simulink model "notch_filters"  (R2014a)
settings: Solver=ode45  StartTime=0.0  StopTime=10.0  RelTol=1e-3
undefined symbols (not defined in the file): A1_notch_cmd, A1_notch_cmd_s, A2_notch_cmd, A2_notch_cmd_s, B1_notch_cmd, B1_notch_cmd_s, B2_notch_cmd, B2_notch_cmd_s, K_notch_cmd, K_notch_cmd_s, sample_time
settings Model: Creator=wmartin  LastModifiedBy=wmartin

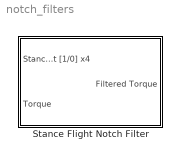
== system notch_filters ==
  Stance Flight Notch Filter : Subsystem

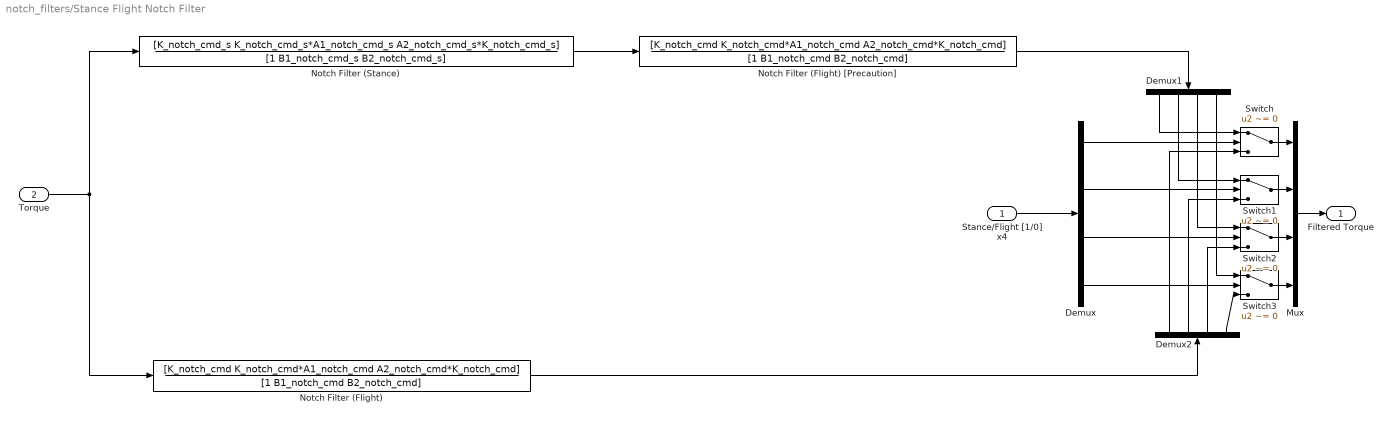
== system notch_filters/Stance Flight Notch Filter ==
  Stance/Flight [1/0] x4 : Inport
  Torque : Inport  Port=2
  Demux : Demux
  Demux1 : Demux
  Demux2 : Demux
  Mux : Mux
  Notch Filter (Flight) : DiscreteTransferFcn  Numerator=[K_notch_cmd K_notch_cmd*A1_notch_cmd A2_notch_cmd*K_notch_cmd]  Denominator=[1 B1_notch_cmd B2_notch_cmd]  SampleTime=sample_time
  Notch Filter (Flight) [Precaution] : DiscreteTransferFcn  Numerator=[K_notch_cmd K_notch_cmd*A1_notch_cmd A2_notch_cmd*K_notch_cmd]  Denominator=[1 B1_notch_cmd B2_notch_cmd]  SampleTime=sample_time
  Notch Filter (Stance) : DiscreteTransferFcn  Numerator=[K_notch_cmd_s K_notch_cmd_s*A1_notch_cmd_s A2_notch_cmd_s*K_notch_cmd_s]  Denominator=[1 B1_notch_cmd_s B2_notch_cmd_s]  SampleTime=sample_time
  Switch{,1..3} (4 alike) : Switch  Criteria=u2 ~= 0
  Filtered Torque : Outport
  wires:
  Notch Filter (Flight) [Precaution]/1 -> Demux1/1
  Demux2/1 -> Switch/3
  Demux2/2 -> Switch1/3
  Demux2/3 -> Switch2/3
  Demux2/4 -> Switch3/3
  Demux1/4 -> Switch3/1
  Demux1/3 -> Switch2/1
  Demux1/2 -> Switch1/1
  Demux1/1 -> Switch/1
  Notch Filter (Stance)/1 -> Notch Filter (Flight) [Precaution]/1
  Demux/1 -> Switch/2
  Switch/1 -> Mux/1
  Mux/1 -> Filtered Torque/1
  Stance/Flight [1/0] x4/1 -> Demux/1
  Switch3/1 -> Mux/4
  Switch2/1 -> Mux/3
  Switch1/1 -> Mux/2
  Demux/2 -> Switch1/2
  Demux/3 -> Switch2/2
  Demux/4 -> Switch3/2
  Notch Filter (Flight)/1 -> Demux2/1
  Torque/1 -> Notch Filter (Stance)/1, Notch Filter (Flight)/1
